simulink model "gal_lib"  (R2016b)
settings: Solver=ode45  StartTime=0.0  StopTime=10.0  RelTol=1e-3  EnableMultiTasking=on
undefined symbols (not defined in the file or in its folder): DiscIntNeverNeededParam
settings Model: Creator=romain  LastModifiedBy=hbourbou
settings DataIOCC: LimitDataPoints=on  SaveFormat=Array  SignalLoggingSaveFormat=ModelDataLogs
settings OptimizationCC: ExpressionDepthLimit=2147483647  LifeSpan=inf
settings DebuggingCC: UnderspecifiedInitializationDetection=Classic  MergeDetectMultiDrivingBlocksExec=none  SolverPrmCheckMsg=warning  FcnCallInpInsideContextMsg=warning  StateNameClashWarn=warning  SFUnexpectedBacktrackingDiag=warning  SFNoUnconditionalDefaultTransitionDiag=warning  SFExecutionAtInitializationDiag=none
settings HardwareCC: ProdBitPerPointer=32  ProdBitPerSizeT=32  ProdBitPerPtrDiffT=32  ProdLargestAtomicFloat=None  ProdIntDivRoundTo=Undefined  ProdEndianess=Unspecified  ProdWordSize=32  ProdHWDeviceType=32-bit Generic
settings ModelReferenceCC: PropagateSignalLabelsOutOfModel=off
settings GRTTargetCC: TargetLangStandard=C89/C90 (ANSI)  GeneratePreprocessorConditionals=Disable all
settings ConfigComp: CovMetricSettings=dw  CovHtmlReporting=on  CovSaveCumulativeToWorkspaceVar=on  CovSaveSingleToWorkspaceVar=on  CovExternalEMLEnable=off  CovSFcnEnable=off

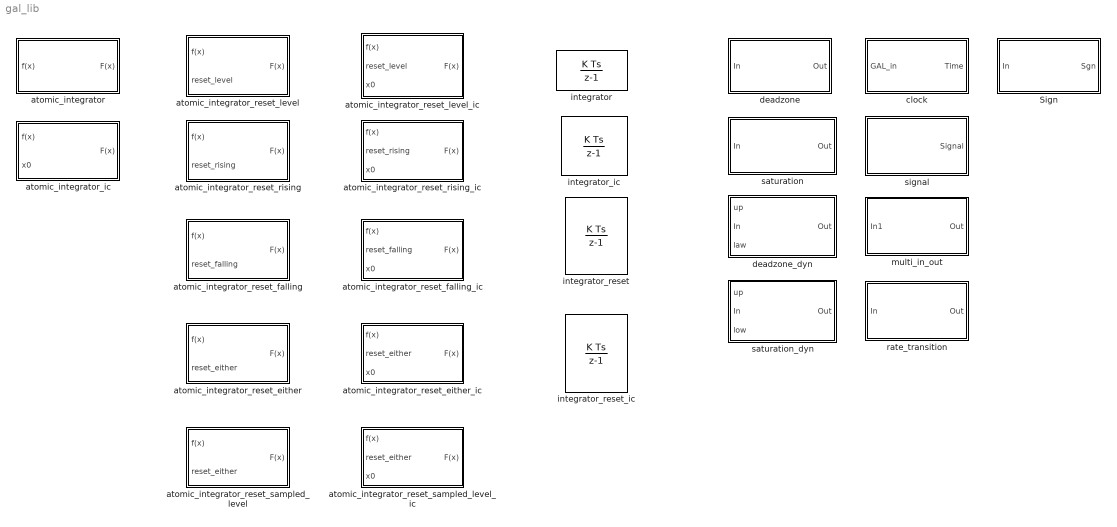
== system gal_lib ==
  Sign : Subsystem
  atomic_integrator : Subsystem
  atomic_integrator_ic : Subsystem
  atomic_integrator_reset_either : Subsystem
  atomic_integrator_reset_either_ic : Subsystem
  atomic_integrator_reset_falling : Subsystem
  atomic_integrator_reset_falling_ic : Subsystem
  atomic_integrator_reset_level : Subsystem
  atomic_integrator_reset_level_ic : Subsystem
  atomic_integrator_reset_rising : Subsystem
  atomic_integrator_reset_rising_ic : Subsystem
  atomic_integrator_reset_sampled_level : Subsystem
  atomic_integrator_reset_sampled_level_ic : Subsystem
  clock : Subsystem
  deadzone : Subsystem
  deadzone_dyn : Subsystem
  integrator : DiscreteIntegrator  InitialConditionSetting=State (most efficient)  SampleTime=-1  ICPrevOutput=DiscIntNeverNeededParam  ICPrevScaledInput=DiscIntNeverNeededParam
  integrator_ic : DiscreteIntegrator  InitialConditionSource=external  InitialConditionSetting=State (most efficient)  SampleTime=-1  ICPrevOutput=DiscIntNeverNeededParam  ICPrevScaledInput=DiscIntNeverNeededParam
  integrator_reset : DiscreteIntegrator  ExternalReset=level  InitialConditionSetting=State (most efficient)  SampleTime=-1  ICPrevOutput=DiscIntNeverNeededParam  ICPrevScaledInput=DiscIntNeverNeededParam
  integrator_reset_ic : DiscreteIntegrator  ExternalReset=level  InitialConditionSource=external  InitialConditionSetting=State (most efficient)  SampleTime=-1  ICPrevOutput=DiscIntNeverNeededParam  ICPrevScaledInput=DiscIntNeverNeededParam
  multi_in_out : Subsystem
  rate_transition : Subsystem
  saturation : Subsystem
  saturation_dyn : Subsystem
  signal : Subsystem

== system gal_lib/Sign ==
  In : Inport
  Constant : Constant  Value=0
  Negative : Constant  Value=-1
  Positive : RelationalOperator  OutDataTypeStr=boolean  RndMeth=Nearest
  Product : Product
  Sum : Sum  Inputs=|++
  not : Logic  Operator=NOT  AllPortsSameDT=off  OutDataTypeStr=boolean
  Sgn : Outport
  wires:
  Constant/1 -> Positive/2
  Sum/1 -> Sgn/1
  Positive/1 -> not/1, Sum/1
  Product/1 -> Sum/2
  Negative/1 -> Product/2
  not/1 -> Product/1
  In/1 -> Positive/1

== system gal_lib/atomic_integrator ==
  f(x) : Inport
  Sample : Gain
  Sum1 : Sum  RequirementInfo={} %GIDa_1d0e93c1_c81a_427d_b24f_cd508f20574b  Inputs=|++
  UnitDelay : UnitDelay  SampleTime=-1
  F(x) : Outport  RequirementInfo={} %GIDa_241d60ba_26b3_49cd_87c7_71748018a914
  wires:
  f(x)/1 -> Sample/1
  UnitDelay/1 -> Sum1/2, F(x)/1
  Sum1/1 -> UnitDelay/1
  Sample/1 -> Sum1/1

== system gal_lib/atomic_integrator_ic ==
  f(x) : Inport
  x0 : Inport  Port=2
  Constant : Constant  Value=0.0  SampleTime=-1
  Product : Product  RndMeth=Zero
  Sample : Gain
  Sum1 : Sum  RequirementInfo={} %GIDa_0d3bcb92_773f_4637_b219_66f0f73283a5  Inputs=|++
  Sum2 : Sum  RequirementInfo={} %GIDa_b356f1af_8a21_416f_a92b_dc7a4aee2a82  Inputs=|++
  Sum3 : Sum  RequirementInfo={} %GIDa_f03eeaaa_8168_4971_8eb8_65abf4816365  Inputs=|++
  UnitDelay : UnitDelay  SampleTime=-1
  UnitDelay1 : UnitDelay  InitialCondition=1  SampleTime=-1
  F(x) : Outport  RequirementInfo={} %GIDa_820f158c_b2af_4fa0_92e0_7d6557d003ca
  wires:
  Sum1/1 -> UnitDelay/1
  Sample/1 -> Sum1/1
  UnitDelay/1 -> Sum3/1, Sum2/1
  Sum2/1 -> Sum1/2
  Product/1 -> Sum3/2, Sum2/2
  UnitDelay1/1 -> Product/2
  Constant/1 -> UnitDelay1/1
  f(x)/1 -> Sample/1
  x0/1 -> Product/1
  Sum3/1 -> F(x)/1

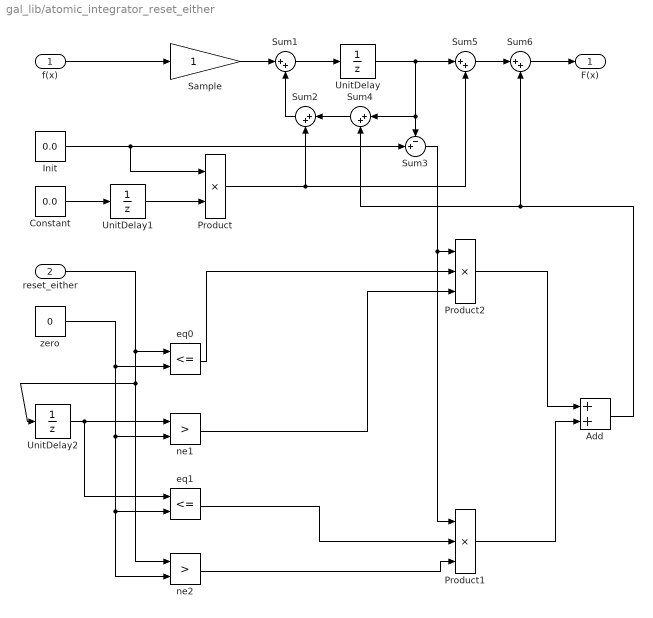
== system gal_lib/atomic_integrator_reset_either ==
  f(x) : Inport
  reset_either : Inport  Port=2
  Add : Sum
  Constant : Constant  Value=0.0  SampleTime=-1
  Init : Constant  Value=0.0  SampleTime=-1
  Product : Product  RndMeth=Zero
  Product1 : Product  Inputs=3  RndMeth=Zero
  Product2 : Product  Inputs=3  RndMeth=Zero
  Sample : Gain
  Sum1 : Sum  RequirementInfo={} %GIDa_c90000cd_84fe_44f5_ade4_911afd7173a7  Inputs=|++
  Sum2 : Sum  RequirementInfo={} %GIDa_2053e7eb_c75e_48ba_9adb_812b1fbc5013  Inputs=|++
  Sum3 : Sum  RequirementInfo={} %GIDa_bd080ba1_c316_49c2_ae04_79ff0a15afab  Inputs=-+|
  Sum4 : Sum  RequirementInfo={} %GIDa_4477bd93_96bf_47a4_a9a6_db7c5459da1e  Inputs=|++
  Sum5 : Sum  RequirementInfo={} %GIDa_0ea36924_be71_4753_b494_f1b9eb5631bc  Inputs=|++
  Sum6 : Sum  RequirementInfo={} %GIDa_4cfeb9ab_3838_42f7_8cb8_15764fc266c5  Inputs=|++
  UnitDelay : UnitDelay  SampleTime=-1
  UnitDelay1 : UnitDelay  InitialCondition=1  SampleTime=-1
  UnitDelay2 : UnitDelay  SampleTime=-1
  eq0 : RelationalOperator  Operator=<=  OutDataTypeStr=boolean  RndMeth=Nearest
  eq1 : RelationalOperator  Operator=<=  OutDataTypeStr=boolean  RndMeth=Nearest
  ne1 : RelationalOperator  Operator=>  OutDataTypeStr=boolean  RndMeth=Nearest
  ne2 : RelationalOperator  Operator=>  OutDataTypeStr=boolean  RndMeth=Nearest
  zero : Constant  Value=0  SampleTime=-1
  F(x) : Outport  RequirementInfo={} %GIDa_cfaa1c84_2887_4b53_9573_dd5665294e9c
  wires:
  Sum1/1 -> UnitDelay/1
  Sample/1 -> Sum1/1
  UnitDelay/1 -> Sum5/1, Sum3/1, Sum4/1
  Sum2/1 -> Sum1/2
  Product/1 -> Sum5/2, Sum2/2
  UnitDelay1/1 -> Product/2
  Constant/1 -> UnitDelay1/1
  Init/1 -> Product/1, Sum3/2
  Sum4/1 -> Sum2/1
  Add/1 -> Sum6/2, Sum4/2
  f(x)/1 -> Sample/1
  Sum5/1 -> Sum6/1
  Sum6/1 -> F(x)/1
  ne1/1 -> Product2/3
  eq0/1 -> Product2/2
  UnitDelay2/1 -> eq1/1, ne1/1
  reset_either/1 -> ne2/1, UnitDelay2/1, eq0/1
  Sum3/1 -> Product1/1, Product2/1
  zero/1 -> ne2/2, eq1/2, ne1/2, eq0/2
  ne2/1 -> Product1/3
  eq1/1 -> Product1/2
  Product1/1 -> Add/2
  Product2/1 -> Add/1

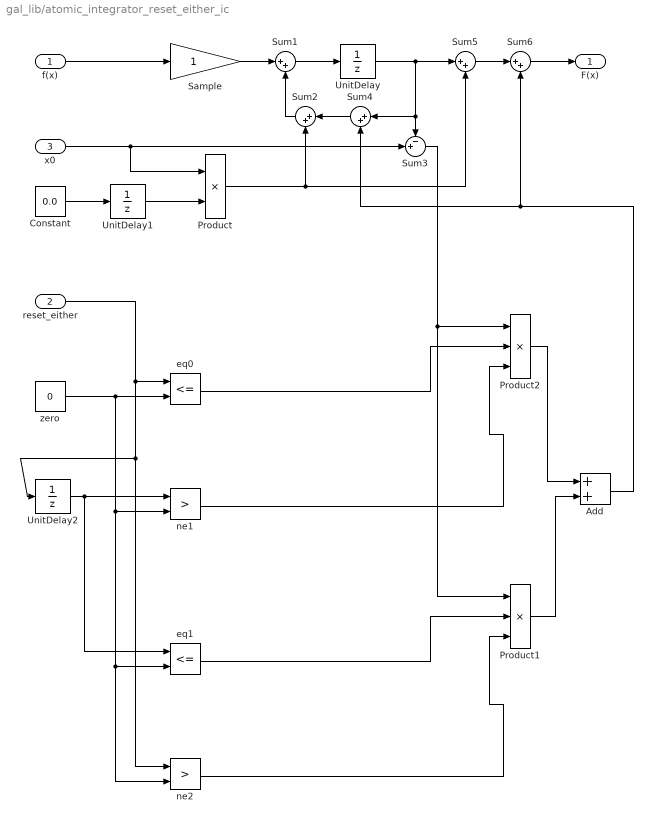
== system gal_lib/atomic_integrator_reset_either_ic ==
  f(x) : Inport
  reset_either : Inport  Port=2
  x0 : Inport  Port=3
  Add : Sum
  Constant : Constant  Value=0.0  SampleTime=-1
  Product : Product  RndMeth=Zero
  Product1 : Product  Inputs=3  RndMeth=Zero
  Product2 : Product  Inputs=3  RndMeth=Zero
  Sample : Gain
  Sum1 : Sum  RequirementInfo={} %GIDa_9e821f1b_e516_466e_acf0_75c1e23ed9e4  Inputs=|++
  Sum2 : Sum  RequirementInfo={} %GIDa_1d26f1e6_1150_4466_ab63_56387d69b272  Inputs=|++
  Sum3 : Sum  RequirementInfo={} %GIDa_6b061376_43f1_4b02_a3e7_bf099b0ee821  Inputs=-+|
  Sum4 : Sum  RequirementInfo={} %GIDa_6b5046c0_ef4a_4df2_bd34_831b7776c08d  Inputs=|++
  Sum5 : Sum  RequirementInfo={} %GIDa_4387a0df_bce6_49fb_a1e2_9ea06a564bd5  Inputs=|++
  Sum6 : Sum  RequirementInfo={} %GIDa_2fb3da95_6082_4606_b8d6_1230bbf90d40  Inputs=|++
  UnitDelay : UnitDelay  SampleTime=-1
  UnitDelay1 : UnitDelay  InitialCondition=1  SampleTime=-1
  UnitDelay2 : UnitDelay  SampleTime=-1
  eq0 : RelationalOperator  Operator=<=  OutDataTypeStr=boolean  RndMeth=Nearest
  eq1 : RelationalOperator  Operator=<=  OutDataTypeStr=boolean  RndMeth=Nearest
  ne1 : RelationalOperator  Operator=>  OutDataTypeStr=boolean  RndMeth=Nearest
  ne2 : RelationalOperator  Operator=>  OutDataTypeStr=boolean  RndMeth=Nearest
  zero : Constant  Value=0  SampleTime=-1
  F(x) : Outport  RequirementInfo={} %GIDa_541e8380_bd89_4557_8859_4ce41a10d526
  wires:
  Sum1/1 -> UnitDelay/1
  Sample/1 -> Sum1/1
  UnitDelay/1 -> Sum5/1, Sum3/1, Sum4/1
  Sum2/1 -> Sum1/2
  Product/1 -> Sum5/2, Sum2/2
  UnitDelay1/1 -> Product/2
  Constant/1 -> UnitDelay1/1
  x0/1 -> Product/1, Sum3/2
  Sum4/1 -> Sum2/1
  Add/1 -> Sum6/2, Sum4/2
  f(x)/1 -> Sample/1
  Sum5/1 -> Sum6/1
  Sum6/1 -> F(x)/1
  ne1/1 -> Product2/3
  eq0/1 -> Product2/2
  UnitDelay2/1 -> eq1/1, ne1/1
  reset_either/1 -> ne2/1, UnitDelay2/1, eq0/1
  Sum3/1 -> Product1/1, Product2/1
  zero/1 -> ne2/2, eq1/2, ne1/2, eq0/2
  ne2/1 -> Product1/3
  eq1/1 -> Product1/2
  Product1/1 -> Add/2
  Product2/1 -> Add/1

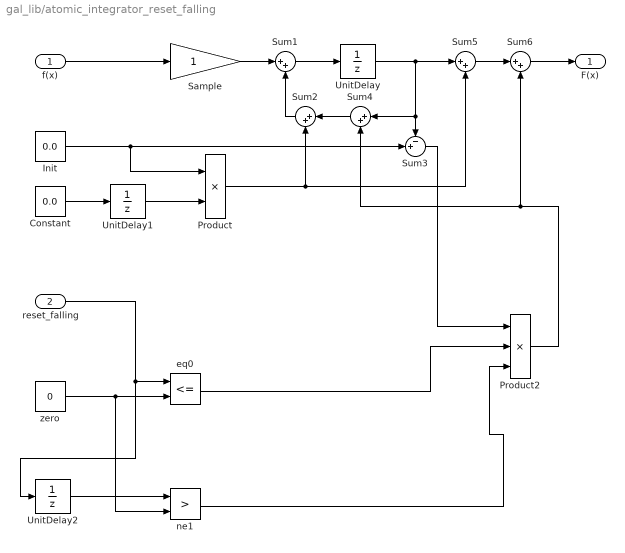
== system gal_lib/atomic_integrator_reset_falling ==
  f(x) : Inport
  reset_falling : Inport  Port=2
  Constant : Constant  Value=0.0  SampleTime=-1
  Init : Constant  Value=0.0  SampleTime=-1
  Product : Product  RndMeth=Zero
  Product2 : Product  Inputs=3  RndMeth=Zero
  Sample : Gain
  Sum1 : Sum  RequirementInfo={} %GIDa_ceed02f4_b646_4b17_81c3_c90ae6f7c25a  Inputs=|++
  Sum2 : Sum  RequirementInfo={} %GIDa_2c9930eb_c170_42dc_9f49_863ebab72455  Inputs=|++
  Sum3 : Sum  RequirementInfo={} %GIDa_8aaf7457_7bef_4eaf_9a24_62e50a4b80c0  Inputs=-+|
  Sum4 : Sum  RequirementInfo={} %GIDa_b8a9049d_81f5_4343_91da_8dab8b3be774  Inputs=|++
  Sum5 : Sum  RequirementInfo={} %GIDa_ef8de264_14a2_4486_98b8_7171205cf833  Inputs=|++
  Sum6 : Sum  RequirementInfo={} %GIDa_5504c618_9948_42d2_9001_5c5c4996b6b8  Inputs=|++
  UnitDelay : UnitDelay  SampleTime=-1
  UnitDelay1 : UnitDelay  InitialCondition=1  SampleTime=-1
  UnitDelay2 : UnitDelay  SampleTime=-1
  eq0 : RelationalOperator  Operator=<=  OutDataTypeStr=boolean  RndMeth=Nearest
  ne1 : RelationalOperator  Operator=>  OutDataTypeStr=boolean  RndMeth=Nearest
  zero : Constant  Value=0  SampleTime=-1
  F(x) : Outport  RequirementInfo={} %GIDa_c20874c0_695c_473c_a690_5fd105ebf643
  wires:
  Sum1/1 -> UnitDelay/1
  Sample/1 -> Sum1/1
  UnitDelay/1 -> Sum5/1, Sum3/1, Sum4/1
  Sum2/1 -> Sum1/2
  Product/1 -> Sum5/2, Sum2/2
  UnitDelay1/1 -> Product/2
  Constant/1 -> UnitDelay1/1
  Init/1 -> Product/1, Sum3/2
  reset_falling/1 -> UnitDelay2/1, eq0/1
  UnitDelay2/1 -> ne1/1
  Sum3/1 -> Product2/1
  zero/1 -> ne1/2, eq0/2
  Sum4/1 -> Sum2/1
  Product2/1 -> Sum6/2, Sum4/2
  f(x)/1 -> Sample/1
  Sum5/1 -> Sum6/1
  Sum6/1 -> F(x)/1
  ne1/1 -> Product2/3
  eq0/1 -> Product2/2

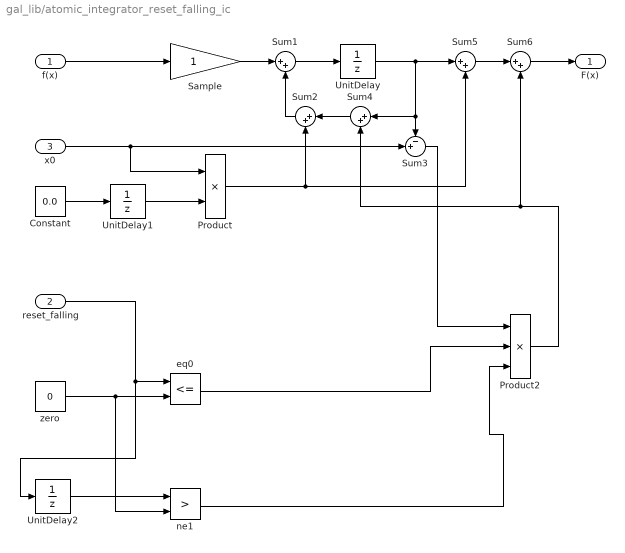
== system gal_lib/atomic_integrator_reset_falling_ic ==
  f(x) : Inport
  reset_falling : Inport  Port=2
  x0 : Inport  Port=3
  Constant : Constant  Value=0.0  SampleTime=-1
  Product : Product  RndMeth=Zero
  Product2 : Product  Inputs=3  RndMeth=Zero
  Sample : Gain
  Sum1 : Sum  RequirementInfo={} %GIDa_afa7aa58_6ac8_4a99_a2f6_5db3c665a659  Inputs=|++
  Sum2 : Sum  RequirementInfo={} %GIDa_5d02d0d7_397f_49ee_840a_e5493da23653  Inputs=|++
  Sum3 : Sum  RequirementInfo={} %GIDa_9a235657_d9ed_4975_a89b_8ee43c6b1924  Inputs=-+|
  Sum4 : Sum  RequirementInfo={} %GIDa_b02cfb3f_81bc_4021_a87b_303b4d71b83f  Inputs=|++
  Sum5 : Sum  RequirementInfo={} %GIDa_7393fc60_e32d_4961_9298_92576b91d4f2  Inputs=|++
  Sum6 : Sum  RequirementInfo={} %GIDa_ca0f2e15_1d0b_4539_926b_34d87c1fd80b  Inputs=|++
  UnitDelay : UnitDelay  SampleTime=-1
  UnitDelay1 : UnitDelay  InitialCondition=1  SampleTime=-1
  UnitDelay2 : UnitDelay  SampleTime=-1
  eq0 : RelationalOperator  Operator=<=  OutDataTypeStr=boolean  RndMeth=Nearest
  ne1 : RelationalOperator  Operator=>  OutDataTypeStr=boolean  RndMeth=Nearest
  zero : Constant  Value=0  SampleTime=-1
  F(x) : Outport  RequirementInfo={} %GIDa_b98a8534_1fa1_40a3_974b_5a40ac934f52
  wires:
  Sum1/1 -> UnitDelay/1
  Sample/1 -> Sum1/1
  UnitDelay/1 -> Sum5/1, Sum3/1, Sum4/1
  Sum2/1 -> Sum1/2
  Product/1 -> Sum5/2, Sum2/2
  UnitDelay1/1 -> Product/2
  Constant/1 -> UnitDelay1/1
  x0/1 -> Product/1, Sum3/2
  reset_falling/1 -> UnitDelay2/1, eq0/1
  UnitDelay2/1 -> ne1/1
  Sum3/1 -> Product2/1
  zero/1 -> ne1/2, eq0/2
  Sum4/1 -> Sum2/1
  Product2/1 -> Sum6/2, Sum4/2
  f(x)/1 -> Sample/1
  Sum5/1 -> Sum6/1
  Sum6/1 -> F(x)/1
  ne1/1 -> Product2/3
  eq0/1 -> Product2/2

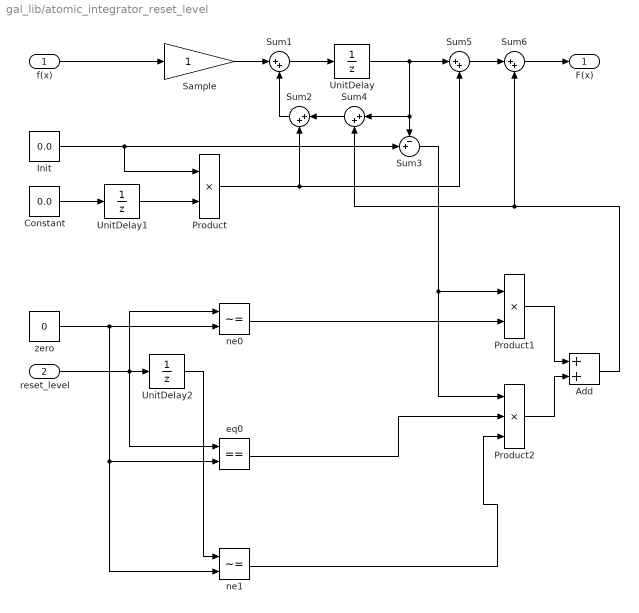
== system gal_lib/atomic_integrator_reset_level ==
  f(x) : Inport
  reset_level : Inport  Port=2
  Add : Sum
  Constant : Constant  Value=0.0  SampleTime=-1
  Init : Constant  Value=0.0  SampleTime=-1
  Product : Product  RndMeth=Zero
  Product1 : Product  RndMeth=Zero
  Product2 : Product  Inputs=3  RndMeth=Zero
  Sample : Gain
  Sum1 : Sum  RequirementInfo={} %GIDa_6b8dd02c_ed84_491d_8ca1_414745e718b3  Inputs=|++
  Sum2 : Sum  RequirementInfo={} %GIDa_04812949_52f8_48ef_be12_aa99c4178e48  Inputs=|++
  Sum3 : Sum  RequirementInfo={} %GIDa_c4dd746e_a8e5_4819_9715_3704ea350af1  Inputs=-+|
  Sum4 : Sum  RequirementInfo={} %GIDa_4f2ce1fb_aa98_40be_84b1_9d8ba4aa16cb  Inputs=|++
  Sum5 : Sum  RequirementInfo={} %GIDa_90db90d1_07e4_4b15_81a3_2d4e5b29a331  Inputs=|++
  Sum6 : Sum  RequirementInfo={} %GIDa_6ad4eec2_af0a_4cc8_ae09_44e1d10623ee  Inputs=|++
  UnitDelay : UnitDelay  SampleTime=-1
  UnitDelay1 : UnitDelay  InitialCondition=1  SampleTime=-1
  UnitDelay2 : UnitDelay  SampleTime=-1
  eq0 : RelationalOperator  Operator===  OutDataTypeStr=boolean  RndMeth=Nearest
  ne0 : RelationalOperator  Operator=~=  OutDataTypeStr=boolean  RndMeth=Nearest
  ne1 : RelationalOperator  Operator=~=  OutDataTypeStr=boolean  RndMeth=Nearest
  zero : Constant  Value=0  SampleTime=-1
  F(x) : Outport  RequirementInfo={} %GIDa_506965f9_2139_49c8_8c1a_31ec06dc7a9e
  wires:
  Sum1/1 -> UnitDelay/1
  Sample/1 -> Sum1/1
  UnitDelay/1 -> Sum5/1, Sum3/1, Sum4/1
  Sum2/1 -> Sum1/2
  Product/1 -> Sum5/2, Sum2/2
  UnitDelay1/1 -> Product/2
  Constant/1 -> UnitDelay1/1
  Init/1 -> Product/1, Sum3/2
  reset_level/1 -> UnitDelay2/1, ne0/1, eq0/1
  UnitDelay2/1 -> ne1/1
  Sum3/1 -> Product1/1, Product2/1
  Product1/1 -> Add/1
  Product2/1 -> Add/2
  zero/1 -> ne0/2, ne1/2, eq0/2
  Sum4/1 -> Sum2/1
  Add/1 -> Sum6/2, Sum4/2
  f(x)/1 -> Sample/1
  Sum5/1 -> Sum6/1
  Sum6/1 -> F(x)/1
  ne1/1 -> Product2/3
  eq0/1 -> Product2/2
  ne0/1 -> Product1/2

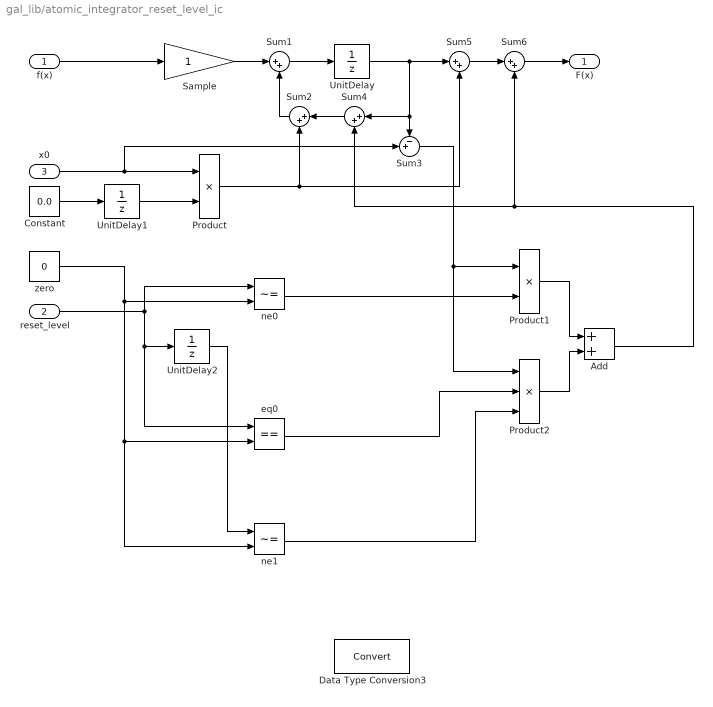
== system gal_lib/atomic_integrator_reset_level_ic ==
  f(x) : Inport
  reset_level : Inport  Port=2
  x0 : Inport  Port=3
  Add : Sum
  Constant : Constant  Value=0.0  SampleTime=-1
  Data Type Conversion3 : DataTypeConversion
  Product : Product  RndMeth=Zero
  Product1 : Product  RndMeth=Zero
  Product2 : Product  Inputs=3  RndMeth=Zero
  Sample : Gain
  Sum1 : Sum  RequirementInfo={} %GIDa_39263520_35b3_4668_b033_635fa337aab2  Inputs=|++
  Sum2 : Sum  RequirementInfo={} %GIDa_ea08176b_e56b_4c76_ac50_8253de048680  Inputs=|++
  Sum3 : Sum  RequirementInfo={} %GIDa_d1f12e52_1972_4ef7_8231_18df582d6b85  Inputs=-+|
  Sum4 : Sum  RequirementInfo={} %GIDa_49fbd192_c8d3_4ed0_9eaf_bd686f0cdf2b  Inputs=|++
  Sum5 : Sum  RequirementInfo={} %GIDa_e801ddfd_c62a_4c6a_9123_2cf222385d60  Inputs=|++
  Sum6 : Sum  RequirementInfo={} %GIDa_e458c5d5_3886_43cb_a694_db902aca0168  Inputs=|++
  UnitDelay : UnitDelay  SampleTime=-1
  UnitDelay1 : UnitDelay  InitialCondition=1  SampleTime=-1
  UnitDelay2 : UnitDelay  SampleTime=-1
  eq0 : RelationalOperator  Operator===  OutDataTypeStr=boolean  RndMeth=Nearest
  ne0 : RelationalOperator  Operator=~=  OutDataTypeStr=boolean  RndMeth=Nearest
  ne1 : RelationalOperator  Operator=~=  OutDataTypeStr=boolean  RndMeth=Nearest
  zero : Constant  Value=0  SampleTime=-1
  F(x) : Outport  RequirementInfo={} %GIDa_a976ad3d_e69d_45ef_9023_54daceffa8ee
  wires:
  Sum1/1 -> UnitDelay/1
  Sample/1 -> Sum1/1
  UnitDelay/1 -> Sum5/1, Sum3/1, Sum4/1
  Sum2/1 -> Sum1/2
  Product/1 -> Sum5/2, Sum2/2
  UnitDelay1/1 -> Product/2
  Constant/1 -> UnitDelay1/1
  x0/1 -> Product/1, Sum3/2
  Sum4/1 -> Sum2/1
  Add/1 -> Sum6/2, Sum4/2
  f(x)/1 -> Sample/1
  Sum5/1 -> Sum6/1
  Sum6/1 -> F(x)/1
  reset_level/1 -> ne0/1, UnitDelay2/1, eq0/1
  UnitDelay2/1 -> ne1/1
  Sum3/1 -> Product1/1, Product2/1
  Product1/1 -> Add/1
  Product2/1 -> Add/2
  zero/1 -> ne0/2, eq0/2, ne1/2
  ne1/1 -> Product2/3
  eq0/1 -> Product2/2
  ne0/1 -> Product1/2
  ? -> Data Type Conversion3/1

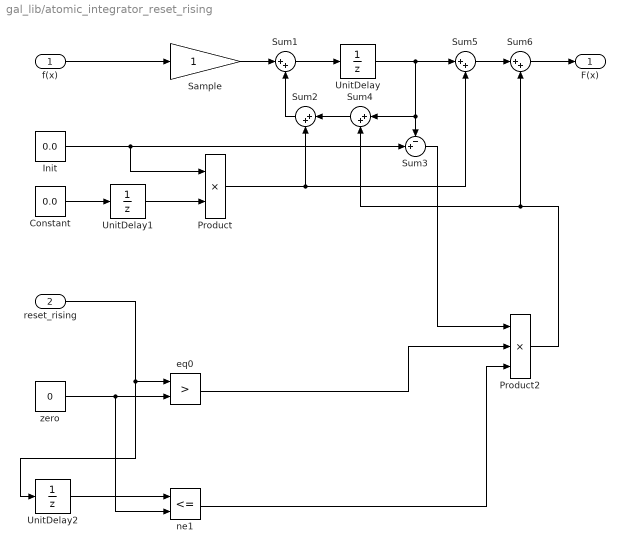
== system gal_lib/atomic_integrator_reset_rising ==
  f(x) : Inport
  reset_rising : Inport  Port=2
  Constant : Constant  Value=0.0  SampleTime=-1
  Init : Constant  Value=0.0  SampleTime=-1
  Product : Product  RndMeth=Zero
  Product2 : Product  Inputs=3  RndMeth=Zero
  Sample : Gain
  Sum1 : Sum  RequirementInfo={} %GIDa_9993d52a_8c8a_4c7a_8b4b_6c1840800012  Inputs=|++
  Sum2 : Sum  RequirementInfo={} %GIDa_96e917c9_0342_401d_bf78_88d75fe2d895  Inputs=|++
  Sum3 : Sum  RequirementInfo={} %GIDa_18cb360c_d0ab_4d80_af14_51f8ea503b64  Inputs=-+|
  Sum4 : Sum  RequirementInfo={} %GIDa_354b7fb4_8889_4ac7_9ccd_c66503c3e688  Inputs=|++
  Sum5 : Sum  RequirementInfo={} %GIDa_ca5c36c8_83bf_4bcb_91ca_a6705132b03a  Inputs=|++
  Sum6 : Sum  RequirementInfo={} %GIDa_11df724f_c1b4_4b1a_b439_ce966be84ded  Inputs=|++
  UnitDelay : UnitDelay  SampleTime=-1
  UnitDelay1 : UnitDelay  InitialCondition=1  SampleTime=-1
  UnitDelay2 : UnitDelay  SampleTime=-1
  eq0 : RelationalOperator  Operator=>  OutDataTypeStr=boolean  RndMeth=Nearest
  ne1 : RelationalOperator  Operator=<=  OutDataTypeStr=boolean  RndMeth=Nearest
  zero : Constant  Value=0  SampleTime=-1
  F(x) : Outport  RequirementInfo={} %GIDa_2bc44fac_f465_4c72_b2f3_7766675caec6
  wires:
  Sum1/1 -> UnitDelay/1
  Sample/1 -> Sum1/1
  UnitDelay/1 -> Sum5/1, Sum3/1, Sum4/1
  Sum2/1 -> Sum1/2
  Product/1 -> Sum5/2, Sum2/2
  UnitDelay1/1 -> Product/2
  Constant/1 -> UnitDelay1/1
  Init/1 -> Product/1, Sum3/2
  reset_rising/1 -> UnitDelay2/1, eq0/1
  UnitDelay2/1 -> ne1/1
  Sum3/1 -> Product2/1
  zero/1 -> ne1/2, eq0/2
  Sum4/1 -> Sum2/1
  Product2/1 -> Sum6/2, Sum4/2
  f(x)/1 -> Sample/1
  Sum5/1 -> Sum6/1
  Sum6/1 -> F(x)/1
  ne1/1 -> Product2/3
  eq0/1 -> Product2/2

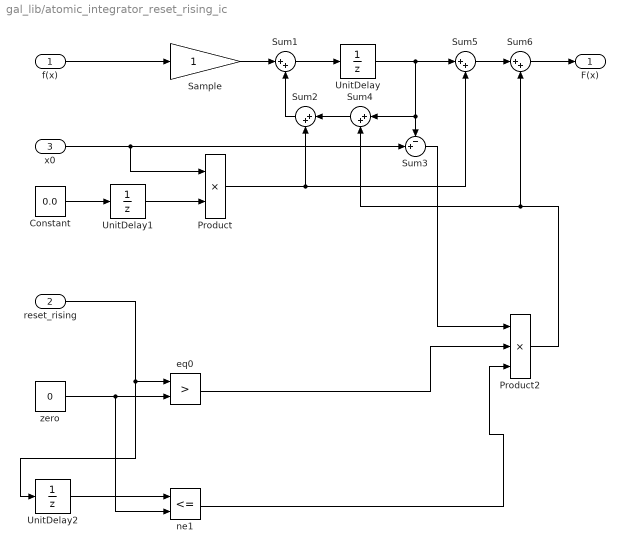
== system gal_lib/atomic_integrator_reset_rising_ic ==
  f(x) : Inport
  reset_rising : Inport  Port=2
  x0 : Inport  Port=3
  Constant : Constant  Value=0.0  SampleTime=-1
  Product : Product  RndMeth=Zero
  Product2 : Product  Inputs=3  RndMeth=Zero
  Sample : Gain
  Sum1 : Sum  RequirementInfo={} %GIDa_df09bd2f_08a1_4e30_937d_22ad7db34251  Inputs=|++
  Sum2 : Sum  RequirementInfo={} %GIDa_7a7abd0d_c3ec_48b6_9598_232a3812a63f  Inputs=|++
  Sum3 : Sum  RequirementInfo={} %GIDa_ea75277b_9f88_4f4f_8248_869eed302a3d  Inputs=-+|
  Sum4 : Sum  RequirementInfo={} %GIDa_7a5ecd27_9a31_4eea_8d29_af3b2ec79a46  Inputs=|++
  Sum5 : Sum  RequirementInfo={} %GIDa_7c862cff_ccc5_427c_863c_0801b5dfac69  Inputs=|++
  Sum6 : Sum  RequirementInfo={} %GIDa_35e457cf_0915_4b3a_8bd2_fd866b05cbe2  Inputs=|++
  UnitDelay : UnitDelay  SampleTime=-1
  UnitDelay1 : UnitDelay  InitialCondition=1  SampleTime=-1
  UnitDelay2 : UnitDelay  SampleTime=-1
  eq0 : RelationalOperator  Operator=>  OutDataTypeStr=boolean  RndMeth=Nearest
  ne1 : RelationalOperator  Operator=<=  OutDataTypeStr=boolean  RndMeth=Nearest
  zero : Constant  Value=0  SampleTime=-1
  F(x) : Outport  RequirementInfo={} %GIDa_4d836b6c_ea13_4b08_91b7_d178a38e74c7
  wires:
  Sum1/1 -> UnitDelay/1
  Sample/1 -> Sum1/1
  UnitDelay/1 -> Sum5/1, Sum3/1, Sum4/1
  Sum2/1 -> Sum1/2
  Product/1 -> Sum5/2, Sum2/2
  UnitDelay1/1 -> Product/2
  Constant/1 -> UnitDelay1/1
  x0/1 -> Product/1, Sum3/2
  reset_rising/1 -> UnitDelay2/1, eq0/1
  UnitDelay2/1 -> ne1/1
  Sum3/1 -> Product2/1
  zero/1 -> ne1/2, eq0/2
  Sum4/1 -> Sum2/1
  Product2/1 -> Sum6/2, Sum4/2
  f(x)/1 -> Sample/1
  Sum5/1 -> Sum6/1
  Sum6/1 -> F(x)/1
  ne1/1 -> Product2/3
  eq0/1 -> Product2/2

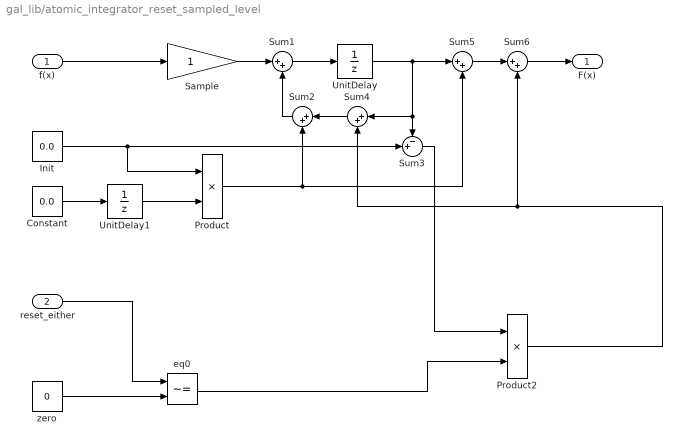
== system gal_lib/atomic_integrator_reset_sampled_level ==
  f(x) : Inport
  reset_either : Inport  Port=2
  Constant : Constant  Value=0.0  SampleTime=-1
  Init : Constant  Value=0.0  SampleTime=-1
  Product : Product  RndMeth=Zero
  Product2 : Product  RndMeth=Zero
  Sample : Gain
  Sum1 : Sum  RequirementInfo={} %GIDa_592c6cfd_0af1_41d4_8684_c3bb0ea8fd73  Inputs=|++
  Sum2 : Sum  RequirementInfo={} %GIDa_39bfe4a1_a06d_418a_8283_b3535e5bfd2d  Inputs=|++
  Sum3 : Sum  RequirementInfo={} %GIDa_83009018_232b_4a41_9a7b_adca44233b6f  Inputs=-+|
  Sum4 : Sum  RequirementInfo={} %GIDa_4dbdeb18_c3af_4957_a8d9_e20d09d68d45  Inputs=|++
  Sum5 : Sum  RequirementInfo={} %GIDa_663ccdaa_985b_434a_8c86_e703105a782d  Inputs=|++
  Sum6 : Sum  RequirementInfo={} %GIDa_be1e523e_a094_4de1_926b_e14ed23618fe  Inputs=|++
  UnitDelay : UnitDelay  SampleTime=-1
  UnitDelay1 : UnitDelay  InitialCondition=1  SampleTime=-1
  eq0 : RelationalOperator  Operator=~=  OutDataTypeStr=boolean  RndMeth=Nearest
  zero : Constant  Value=0  SampleTime=-1
  F(x) : Outport  RequirementInfo={} %GIDa_d7ae9251_2d75_4b46_ad7a_969d90cfa16d
  wires:
  Sum1/1 -> UnitDelay/1
  Sample/1 -> Sum1/1
  UnitDelay/1 -> Sum5/1, Sum3/1, Sum4/1
  Sum2/1 -> Sum1/2
  Product/1 -> Sum5/2, Sum2/2
  UnitDelay1/1 -> Product/2
  Constant/1 -> UnitDelay1/1
  Init/1 -> Product/1, Sum3/2
  Sum4/1 -> Sum2/1
  Product2/1 -> Sum6/2, Sum4/2
  f(x)/1 -> Sample/1
  Sum5/1 -> Sum6/1
  Sum6/1 -> F(x)/1
  eq0/1 -> Product2/2
  reset_either/1 -> eq0/1
  Sum3/1 -> Product2/1
  zero/1 -> eq0/2

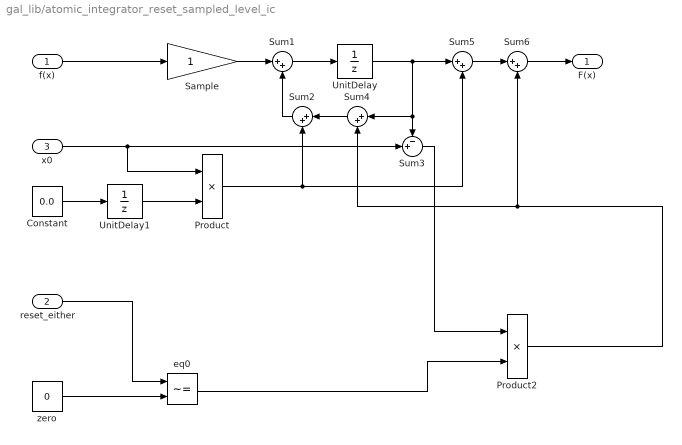
== system gal_lib/atomic_integrator_reset_sampled_level_ic ==
  f(x) : Inport
  reset_either : Inport  Port=2
  x0 : Inport  Port=3
  Constant : Constant  Value=0.0  SampleTime=-1
  Product : Product  RndMeth=Zero
  Product2 : Product  RndMeth=Zero
  Sample : Gain
  Sum1 : Sum  RequirementInfo={} %GIDa_b19d7a44_b07d_464c_bb03_c02893cf317e  Inputs=|++
  Sum2 : Sum  RequirementInfo={} %GIDa_f6236ddb_2de2_4896_8453_b7f30b5b37fc  Inputs=|++
  Sum3 : Sum  RequirementInfo={} %GIDa_a7087afd_81af_4f0f_9cd9_4e98b86ea078  Inputs=-+|
  Sum4 : Sum  RequirementInfo={} %GIDa_2ebdf18f_af1d_4550_8fa5_73384d483a61  Inputs=|++
  Sum5 : Sum  RequirementInfo={} %GIDa_5563d5a4_73b4_4603_9ad5_feea2da0fb03  Inputs=|++
  Sum6 : Sum  RequirementInfo={} %GIDa_cd766a52_da4e_4683_a088_870148817066  Inputs=|++
  UnitDelay : UnitDelay  SampleTime=-1
  UnitDelay1 : UnitDelay  InitialCondition=1  SampleTime=-1
  eq0 : RelationalOperator  Operator=~=  OutDataTypeStr=boolean  RndMeth=Nearest
  zero : Constant  Value=0  SampleTime=-1
  F(x) : Outport  RequirementInfo={} %GIDa_0876e0a5_7196_43e3_b16d_e85d81fafee9
  wires:
  Sum1/1 -> UnitDelay/1
  Sample/1 -> Sum1/1
  UnitDelay/1 -> Sum5/1, Sum3/1, Sum4/1
  Sum2/1 -> Sum1/2
  Product/1 -> Sum5/2, Sum2/2
  UnitDelay1/1 -> Product/2
  Constant/1 -> UnitDelay1/1
  x0/1 -> Product/1, Sum3/2
  Sum4/1 -> Sum2/1
  Product2/1 -> Sum6/2, Sum4/2
  f(x)/1 -> Sample/1
  Sum5/1 -> Sum6/1
  Sum6/1 -> F(x)/1
  eq0/1 -> Product2/2
  reset_either/1 -> eq0/1
  Sum3/1 -> Product2/1
  zero/1 -> eq0/2

== system gal_lib/clock ==
  GAL_in : Inport
  Constant : Constant  SampleTime=Inf
  Sample : Gain
  Sum1 : Sum  RequirementInfo={} %GIDa_75b643fa_a90c_4741_89ed_d97a0d8d6e0d  Inputs=|++
  delay : UnitDelay  SampleTime=-1
  Time : Outport  RequirementInfo={} %GIDa_dc45b9eb_11b9_47b3_ab00_f1590eb2152b
  wires:
  Constant/1 -> Sample/1
  delay/1 -> Sum1/2, Time/1
  Sum1/1 -> delay/1
  Sample/1 -> Sum1/1

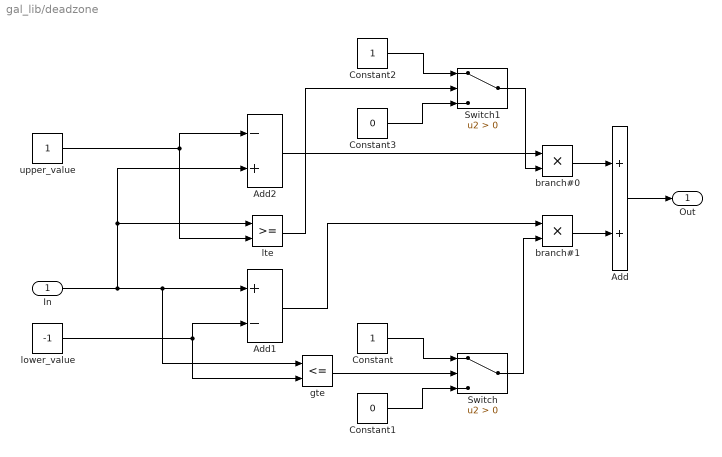
== system gal_lib/deadzone ==
  In : Inport
  Add : Sum
  Add1 : Sum  Inputs=+-
  Add2 : Sum  Inputs=-+
  Constant : Constant
  Constant1 : Constant  Value=0
  Constant2 : Constant
  Constant3 : Constant  Value=0
  Switch : Switch  Criteria=u2 > Threshold
  Switch1 : Switch  Criteria=u2 > Threshold
  branch#0 : Product  RndMeth=Zero
  branch#1 : Product  RndMeth=Zero
  gte : RelationalOperator  Operator=<=  OutDataTypeStr=boolean  RndMeth=Nearest
  lower_value : Constant  Value=-1  SampleTime=-1
  lte : RelationalOperator  OutDataTypeStr=boolean  RndMeth=Nearest
  upper_value : Constant  SampleTime=-1
  Out : Outport
  wires:
  In/1 -> Add1/1, gte/1, Add2/2, lte/1
  lower_value/1 -> Add1/2, gte/2
  Add/1 -> Out/1
  upper_value/1 -> Add2/1, lte/2
  Add2/1 -> branch#0/1
  branch#0/1 -> Add/1
  Add1/1 -> branch#1/1
  gte/1 -> Switch/2
  branch#1/1 -> Add/2
  Constant/1 -> Switch/1
  Constant1/1 -> Switch/3
  Switch/1 -> branch#1/2
  lte/1 -> Switch1/2
  Constant2/1 -> Switch1/1
  Constant3/1 -> Switch1/3
  Switch1/1 -> branch#0/2

== system gal_lib/deadzone_dyn ==
  up : Inport
  In : Inport  Port=2
  law : Inport  Port=3
  Add : Sum
  Add1 : Sum  Inputs=+-
  Add2 : Sum  Inputs=-+
  Constant : Constant
  Constant1 : Constant  Value=0
  Constant2 : Constant
  Constant3 : Constant  Value=0
  Switch : Switch  Criteria=u2 > Threshold
  Switch1 : Switch  Criteria=u2 > Threshold
  branch#0 : Product  RndMeth=Zero
  branch#1 : Product  RndMeth=Zero
  gte : RelationalOperator  Operator=<=  OutDataTypeStr=boolean  RndMeth=Nearest
  lte : RelationalOperator  OutDataTypeStr=boolean  RndMeth=Nearest
  Out : Outport
  wires:
  In/1 -> Add1/1, gte/1, Add2/2, lte/1
  law/1 -> Add1/2, gte/2
  Add/1 -> Out/1
  up/1 -> Add2/1, lte/2
  Add2/1 -> branch#0/1
  branch#0/1 -> Add/1
  Add1/1 -> branch#1/1
  gte/1 -> Switch/2
  branch#1/1 -> Add/2
  Constant/1 -> Switch/1
  Constant1/1 -> Switch/3
  Switch/1 -> branch#1/2
  lte/1 -> Switch1/2
  Constant2/1 -> Switch1/1
  Constant3/1 -> Switch1/3
  Switch1/1 -> branch#0/2

== system gal_lib/multi_in_out ==
  In1 : Inport
  Demux : Demux  Outputs=2
  Mux : Mux  Inputs=2
  multi_block : Subsystem
  Out : Outport  RequirementInfo={} %GIDa_0ffe225d_c3ba_42a6_8663_21506e49c7a0
  wires:
  Mux/1 -> Out/1
  In1/1 -> Demux/1

== system gal_lib/rate_transition ==
  In : Inport
  Constant : Constant  Value=0.0  SampleTime=-1
  Init : Constant  Value=0.0  SampleTime=-1
  Product : Product  RndMeth=Zero
  Sum : Sum  Inputs=|++
  UnitDelay : UnitDelay  InitialCondition=1  SampleTime=-1
  Out : Outport  RequirementInfo={} %GIDa_abf0c760_2bd7_4265_a845_7e43c44d726d
  wires:
  Product/1 -> Sum/2
  UnitDelay/1 -> Product/2
  Constant/1 -> UnitDelay/1
  In/1 -> Sum/1
  Sum/1 -> Out/1
  Init/1 -> Product/1

== system gal_lib/saturation ==
  In : Inport
  lower : MinMax  Function=max  Inputs=2
  lower_limit : Constant  Value=-1.0  SampleTime=-1
  upper : MinMax  Inputs=2
  upper_limit : Constant  Value=1.0  SampleTime=-1
  Out : Outport
  wires:
  upper_limit/1 -> upper/1
  upper/1 -> lower/1
  lower_limit/1 -> lower/2
  In/1 -> upper/2
  lower/1 -> Out/1

== system gal_lib/saturation_dyn ==
  up : Inport
  In : Inport  Port=2
  low : Inport  Port=3
  lower : MinMax  Function=max  Inputs=2
  upper : MinMax  Inputs=2
  Out : Outport
  wires:
  up/1 -> upper/1
  upper/1 -> lower/1
  low/1 -> lower/2
  In/1 -> upper/2
  lower/1 -> Out/1

== system gal_lib/signal ==
  Constant : Constant
  Sample : Gain
  Sum1 : Sum  RequirementInfo={} %GIDa_ad1be89b_5ea6_4ca7_b97b_97c05bfa813c  Inputs=|++
  delay : UnitDelay  SampleTime=-1
  signal_generator : Subsystem
  Signal : Outport  RequirementInfo={} %GIDa_ed73f4d3_9598_42a3_8120_8d58418c8ab4
  wires:
  signal_generator/1(Out1) -> Signal/1
  delay/1 -> signal_generator/1(In1), Sum1/2
  Constant/1 -> Sample/1
  Sum1/1 -> delay/1
  Sample/1 -> Sum1/1

== system gal_lib/multi_in_out/multi_block ==
  In1 : Inport
  Out1 : Outport
  wires:
  In1/1 -> Out1/1

== system gal_lib/signal/signal_generator ==
  In1 : Inport
  Out1 : Outport
  wires:
  In1/1 -> Out1/1
